simulink model "untitled"  (Simulink 7.8)
settings: Solver=ode45  StartTime=0.0  StopTime=10.0  RelTol=1e-3
libraries: simulink x2
settings Model: Creator=--  LastModifiedBy=--

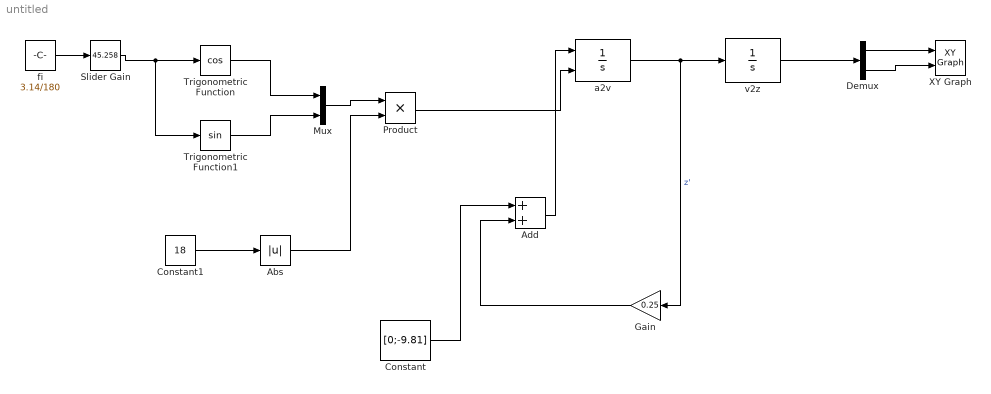
== system untitled ==
  Abs : Abs
  Add : Sum
  Constant : Constant  Value=[0;-9.81]
  Constant1 : Constant  Value=18
  Demux : Demux  Outputs=2
  Gain : Gain  Gain=0.25
  Mux : Mux  Inputs=2
  Product : Product  RndMeth=Zero
  Slider Gain : simulink/Math Operations/Slider Gain  low=0  gain=45.258  high=90
  Trigonometric Function : Trigonometry  Operator=cos
  Trigonometric Function1 : Trigonometry
  XY Graph : simulink/Sinks/XY Graph  xmin=0  xmax=50  ymin=0  ymax=30  st=-1
  a2v : Integrator  InitialConditionSource=external  InitialCondition=[10;10]  UpperSaturationLimit=1  LowerSaturationLimit=0
  fi : Constant  Value=3.14/180
  v2z : Integrator  UpperSaturationLimit=1  LowerSaturationLimit=0
  wires:
  a2v/1 -> v2z/1, Gain/1  "z'"
  Gain/1 -> Add/2
  Constant/1 -> Add/1
  Add/1 -> a2v/1
  v2z/1 -> Demux/1
  Demux/1 -> XY Graph/1
  Demux/2 -> XY Graph/2
  fi/1 -> Slider Gain/1
  Trigonometric Function/1 -> Mux/1
  Trigonometric Function1/1 -> Mux/2
  Mux/1 -> Product/1
  Constant1/1 -> Abs/1
  Abs/1 -> Product/2
  Product/1 -> a2v/2
  Slider Gain/1 -> Trigonometric Function/1, Trigonometric Function1/1
